simulink model "ccsdsLDPCModel"  (R2024a)
settings: Solver=VariableStepAuto  StartTime=0.0  StopTime=simTime  RelTol=1e-3
libraries: dspsrcs4 x4, whdlutilities x2, whdledac x1
settings Model: SimulationMode=accelerator  VariantFading=off  Creator=The MathWorks, Inc.  LastModifiedBy=Anthony
settings SolverCC: MaxZcPerStep=1
settings OptimizationCC: BlockReduction=off  ConditionallyExecuteInputs=off  ReuseModelBlockBuffer=off
settings DebuggingCC: IntegerOverflowMsg=none
settings ModelReferenceCC: EnableRefExpFcnMdlSchedulingChecks=on
settings RTWCC: GPUComputeCapability=3.5  DLArmComputeVersion=19.05

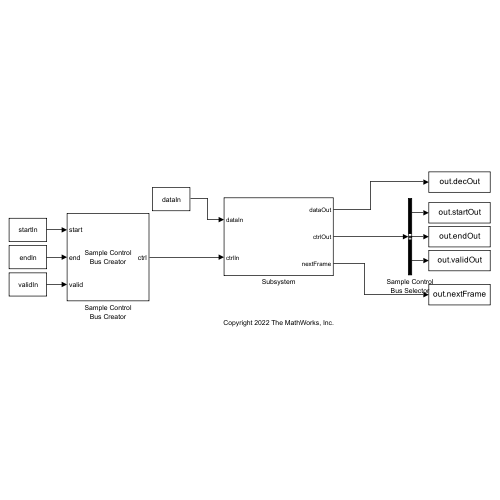
[thumbnail: Simulink's stored preview of the top-level diagram]
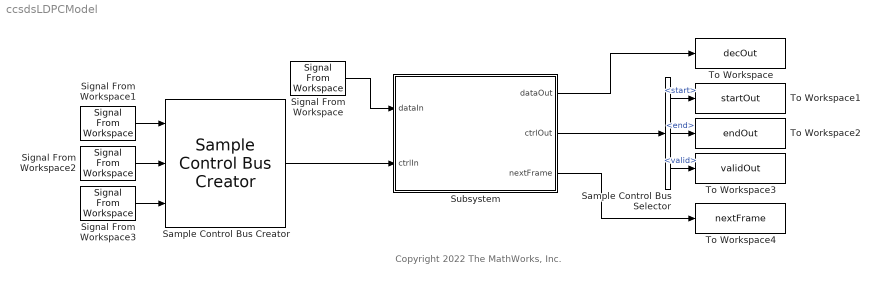
== system ccsdsLDPCModel ==
  note: Copyright 2022 The MathWorks, Inc.
  Sample Control Bus Creator : whdlutilities/Sample Control Bus Creator
  Sample Control Bus Selector : whdlutilities/Sample Control Bus Selector  OutputSignals=start,end,valid
  Signal From Workspace : dspsrcs4/Signal From Workspace  X=dataIn  Ts=1  nsamps=1  OutputAfterFinalValue=Setting to zero  ignoreOrWarnInputAndFrameLengths=off  OutputFrames=off
  Signal From Workspace1 : dspsrcs4/Signal From Workspace  X=startIn  Ts=1  nsamps=1  OutputAfterFinalValue=Setting to zero  ignoreOrWarnInputAndFrameLengths=off  OutputFrames=off
  Signal From Workspace2 : dspsrcs4/Signal From Workspace  X=endIn  Ts=1  nsamps=1  OutputAfterFinalValue=Setting to zero  ignoreOrWarnInputAndFrameLengths=off  OutputFrames=off
  Signal From Workspace3 : dspsrcs4/Signal From Workspace  X=validIn  Ts=1  nsamps=1  OutputAfterFinalValue=Setting to zero  ignoreOrWarnInputAndFrameLengths=off  OutputFrames=off
  Subsystem : Subsystem
  To Workspace : ToWorkspace  VariableName=decOut  SampleTime=-1
  To Workspace1 : ToWorkspace  VariableName=startOut  SampleTime=-1
  To Workspace2 : ToWorkspace  VariableName=endOut  SampleTime=-1
  To Workspace3 : ToWorkspace  VariableName=validOut  SampleTime=-1
  To Workspace4 : ToWorkspace  VariableName=nextFrame  SampleTime=-1
  wires:
  Signal From Workspace1/1 -> Sample Control Bus Creator/1
  Signal From Workspace2/1 -> Sample Control Bus Creator/2
  Signal From Workspace3/1 -> Sample Control Bus Creator/3
  Signal From Workspace/1 -> Subsystem/1(dataIn)
  Sample Control Bus Creator/1 -> Subsystem/2(ctrlIn)
  Subsystem/3(nextFrame) -> To Workspace4/1
  Sample Control Bus Selector/1 -> To Workspace1/1  "<start>"
  Sample Control Bus Selector/2 -> To Workspace2/1  "<end>"
  Subsystem/2(ctrlOut) -> Sample Control Bus Selector/1
  Subsystem/1(dataOut) -> To Workspace/1
  Sample Control Bus Selector/3 -> To Workspace3/1  "<valid>"

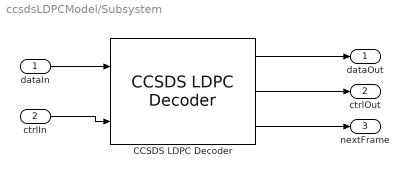
== system ccsdsLDPCModel/Subsystem ==
  dataIn : Inport
  ctrlIn : Inport  Port=2
  CCSDS LDPC Decoder : whdledac/CCSDS LDPC Decoder  LDPCConfiguration=(8160,7136) LDPC  Termination=Max  SpecifyInputs=Property  NumIterations=max_iter  MaxNumIterations=numIter  ParityCheckStatus=off  SimulateUsing=Code generation
  dataOut : Outport
  ctrlOut : Outport  Port=2
  nextFrame : Outport  Port=3
  wires:
  CCSDS LDPC Decoder/1 -> dataOut/1
  dataIn/1 -> CCSDS LDPC Decoder/1
  ctrlIn/1 -> CCSDS LDPC Decoder/2
  CCSDS LDPC Decoder/2 -> ctrlOut/1
  CCSDS LDPC Decoder/3 -> nextFrame/1
